simulink model "ModeleMachineInduction"  (R2022b)
settings: Solver=VariableStepAuto  StartTime=0.0  StopTime=10.0  MaxStep=10e-6  RelTol=1e-3
values from neighbouring files (symbols this model uses):
  fv = 0.08    [MotorDat_MSTPM1 (1).m]    (also in ParamMinduction0.m = 0.137399950871)
  h = 50e-6    (= 5e-05)    [MotorDat_MSTPM1 (1).m]    (also in ParamMinduction0.m; parametres.m = 1e-05)
  J = 0.004    [MotorDat_MSTPM1 (1).m]    (also in ParamMinduction0.m = 0.006; parametres.m = 0.000131)
  k_v = 0.8489    [ParamMinduction0.m]
  lcs_v = 62e-3    (= 0.062)    [ParamMinduction0.m]
  p = 4    [MotorDat_MSTPM1 (1).m]    (also in ParamMinduction0.m = 2)
  Rr_v = 1.8    [ParamMinduction0.m]
  Rs_v = 2.5    [ParamMinduction0.m]
  Tr_v = Lcr_v/Rr_v    (= 0.268333333333)    [ParamMinduction0.m]
  Vmax = 530    [MotorDat_MSTPM1 (1).m]    (also in ParamMinduction0.m = 650; parametres.m = 0.171666666667)
libraries: simulink x1, slpidlib x1
settings Model: Creator=dgrenier  LastModifiedBy=boris
settings DebuggingCC: UnconnectedInputMsg=warning  UnconnectedOutputMsg=warning  UnconnectedLineMsg=warning
settings ModelReferenceCC: EnableRefExpFcnMdlSchedulingChecks=on
settings RTWCC: DLArmComputeVersion=19.05

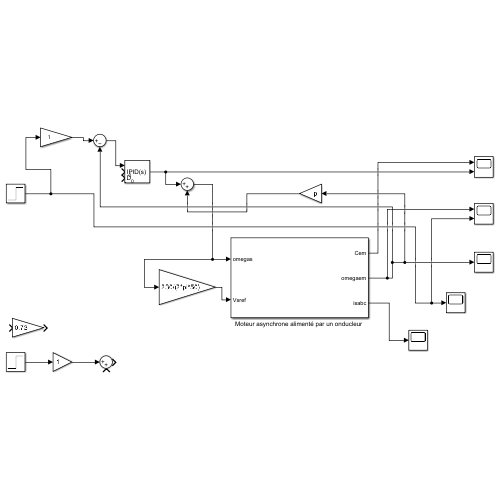
[thumbnail: Simulink's stored preview of the top-level diagram]
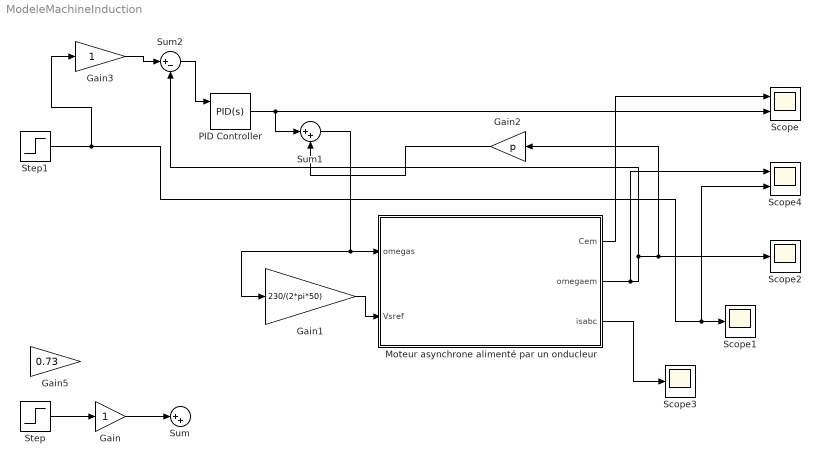
== system ModeleMachineInduction ==
  Gain : Gain
  Gain1 : Gain  Gain=230/(2*pi*50)
  Gain2 : Gain  Gain=p
  Gain3 : Gain
  Gain5 : Gain  Gain=0.73
  "Moteur asynchrone alimenté par un onducleur " : Subsystem
  PID Controller : slpidlib/PID Controller  Controller=PID  Form=Parallel  TimeDomain=Continuous-time  UseExternalTs=off  SampleTime=-1  IntegratorMethod=Forward Euler  FilterMethod=Forward Euler  ControllerParametersSource=internal  P=10  I=1  UseKiTs=off  D=0  N=100  UseFilter=on  TunerSelectOption=Transfer Function Based (PID Tuner App)  InitialConditionSource=external  InitialConditionForIntegrator=0  InitialConditionForFilter=0  DifferentiatorICPrevScaledInput=0  ExternalReset=none  TrackingMode=off  Kt=1  LimitOutput=off  SatLimitsSource=internal  UpperSaturationLimit=inf  LowerSaturationLimit=-inf  LinearizeAsGain=on  AntiWindupMode=none  Kb=1  LimitIntegrator=off  UpperIntegratorSaturationLimit=inf  LowerIntegratorSaturationLimit=-inf  POutMin=[]  POutMax=[]  IOutMin=[]  IOutMax=[]  DOutMin=[]  DOutMax=[]  NOutMin=[]  NOutMax=[]  SumOutMin=[]  SumOutMax=[]  SaturationOutMin=[]  SaturationOutMax=[]  PParamMin=[]  PParamMax=[]  IParamMin=[]  IParamMax=[]  DParamMin=[]  DParamMax=[]  NParamMin=[]  NParamMax=[]  KbParamMin=[]  KbParamMax=[]  KtParamMin=[]  KtParamMax=[]  KbOutMin=[]  KbOutMax=[]  KtOutMin=[]  KtOutMax=[]  IntegratorOutMin=[]  IntegratorOutMax=[]  FilterOutMin=[]  FilterOutMax=[]  SumI1OutMin=[]  SumI1OutMax=[]  SumI2OutMin=[]  SumI2OutMax=[]  SumI3OutMin=[]  SumI3OutMax=[]  SumI4OutMin=[]  SumI4OutMax=[]  SumDOutMin=[]  SumDOutMax=[]  DifferentiatorOutMin=[]  DifferentiatorOutMax=[]  FilterDiffOutCoefMin=[]  FilterDiffOutCoefMax=[]  ReciprocalOutMin=[]  ReciprocalOutMax=[]  SumDenOutMin=[]  SumDenOutMax=[]  SumNumOutMin=[]  SumNumOutMax=[]  DivideOutMin=[]  DivideOutMax=[]  UdiffTsProdOutMin=[]  UdiffTsProdOutMax=[]  NTsProdOutMin=[]  NTsProdOutMax=[]  UintegralTsProdOutMin=[]  UintegralTsProdOutMax=[]  UngainTsProdOutMin=[]  UngainTsProdOutMax=[]  ClampingZeroOutDataTypeStr=Inherit: Inherit via back propagation  ClampingZeroOutMin=[]  ClampingZeroOutMax=[]  FilterDenConstantOutDataTypeStr=Inherit: Inherit via back propagation  FilterDenConstantOutMin=[]  FilterDenConstantOutMax=[]  PCopyOutDataTypeStr=Inherit: Inherit via back propagation  PCopyOutMin=[]  PCopyOutMax=[]  NCopyOutDataTypeStr=Inherit: Inherit via back propagation  NCopyOutMin=[]  NCopyOutMax=[]  IntegratorContinuousStateAttributes=''  IntegratorStateMustResolveToSignalObject=off  IntegratorRTWStateStorageClass=Auto  FilterContinuousStateAttributes=''  FilterStateMustResolveToSignalObject=off  FilterRTWStateStorageClass=Auto  ParallelPVariant=InternalParameters  IdealPVariant=Disabled  IVariant=InternalParameters  DVariant=InternalParameters  IntegratorVariant=Continuous  SatVariant=Disabled  AWVariant=Passthrough  PCopyVariant=Disabled  TRVariant=Disabled  FdbkBlocksVariant=Forward  IdealPFdbkVariant=Disabled  SatFdbkVariant=Disabled  DerivativeFilterVariant=ContFilter  NVariant=InternalParameters  NCopyVariant=Disabled  FilterICVariant=ExternalICs  IntegratorICVariant=ExternalICs  ExternalResetVariant=Disabled  TRSumVariant=Passthrough  SumFdbkVariant=Disabled  SumVariant=Sum_PID  TsampFilterVariant=InternalTs  TsampNgainVariant=Passthrough  TsampIntegralVariant=Passthrough  ExternalSaturationOutDataTypeStr=Inherit: Same as second input
  Scope : Scope  NumInputPorts=2
  Scope1 : Scope
  Scope2 : Scope
  Scope3 : Scope
  Scope4 : Scope  NumInputPorts=2
  Step : Step  SampleTime=0
  Step1 : Step  After=10  SampleTime=1
  Sum : Sum  Inputs=|++
  Sum1 : Sum  Inputs=|++
  Sum2 : Sum  Inputs=|+-
  wires:
  Gain/1 -> Sum/1
  Step/1 -> Gain/1
  Sum1/1 -> Gain1/1, "Moteur asynchrone alimenté par un onducleur "/1(omegas)
  Gain2/1 -> Sum1/2
  "Moteur asynchrone alimenté par un onducleur "/2(omegaem) -> Scope4/1, Scope2/1, Gain2/1, Sum2/2
  "Moteur asynchrone alimenté par un onducleur "/3(isabc) -> Scope3/1
  Gain1/1 -> "Moteur asynchrone alimenté par un onducleur "/2(Vsref)
  Step1/1 -> Scope4/2, Scope1/1, Gain3/1
  Sum2/1 -> PID Controller/1
  Gain3/1 -> Sum2/1
  "Moteur asynchrone alimenté par un onducleur "/1(Cem) -> Scope/1
  PID Controller/1 -> Sum1/1, Scope/2

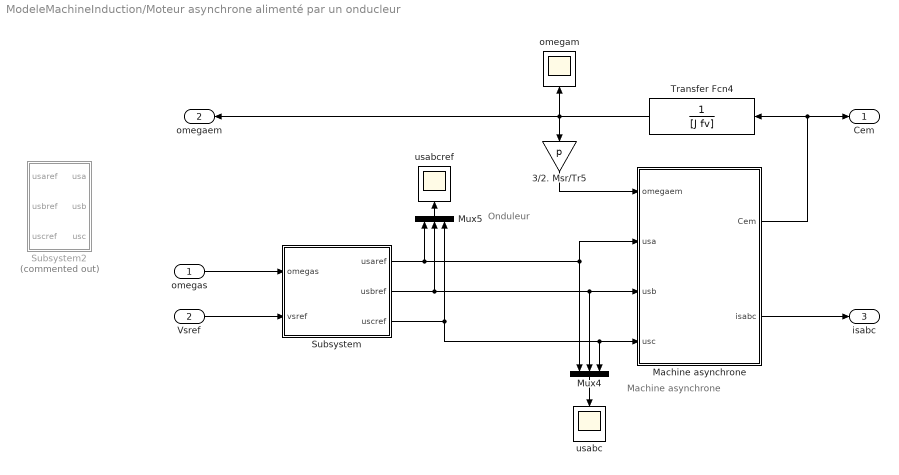
== system ModeleMachineInduction/Moteur asynchrone alimenté par un onducleur  ==
  note: Machine asynchrone
  note: Onduleur
  omegas : Inport
  Vsref : Inport  Port=2
  3/2. Msr/Tr5 : Gain  Gain=p
  Machine asynchrone : Subsystem
  Mux4 : Mux  Inputs=3
  Mux5 : Mux  Inputs=3
  Subsystem : Subsystem
  Subsystem2 : Subsystem  Commented=on
  Transfer Fcn4 : TransferFcn  Denominator=[J fv]
  "omegam " : Scope
  usabc : Scope
  usabcref : Scope
  Cem : Outport
  omegaem : Outport  Port=2
  isabc : Outport  Port=3
  wires:
  omegas/1 -> Subsystem/1(omegas)
  Vsref/1 -> Subsystem/2(vsref)
  Subsystem/3(uscref) -> Machine asynchrone/4(usc), Mux4/3, Mux5/3
  Subsystem/1(usaref) -> Machine asynchrone/2(usa), Mux4/1, Mux5/1
  Mux5/1 -> usabcref/1
  Subsystem/2(usbref) -> Machine asynchrone/3(usb), Mux4/2, Mux5/2
  Mux4/1 -> usabc/1
  Machine asynchrone/1(Cem) -> Cem/1, Transfer Fcn4/1
  Machine asynchrone/2(isabc) -> isabc/1
  3/2. Msr/Tr5/1 -> Machine asynchrone/1(omegaem)
  Transfer Fcn4/1 -> "omegam "/1, 3/2. Msr/Tr5/1, omegaem/1

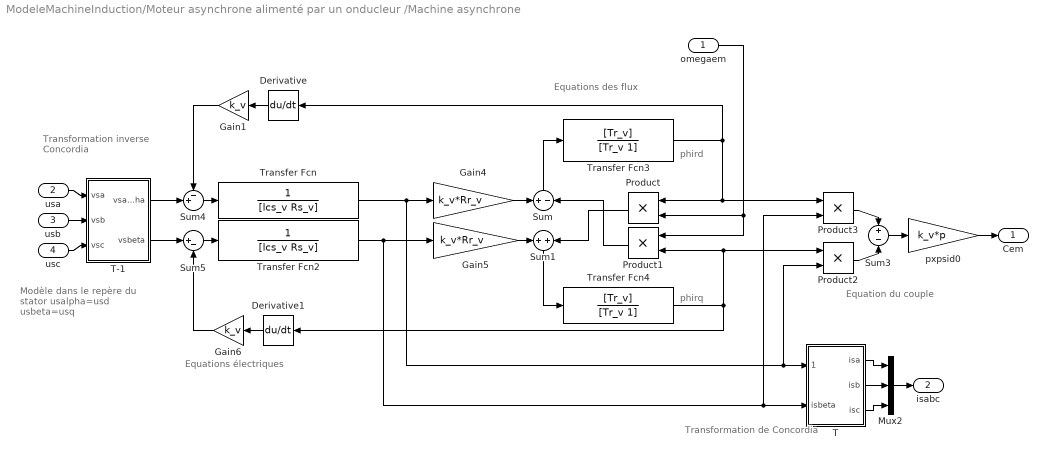
== system ModeleMachineInduction/Moteur asynchrone alimenté par un onducleur /Machine asynchrone ==
  note: Transformation
      | de Concordia
  note: Transformation
      | inverse Concordia
  note: Equation du couple
  note: Equations électriques
  note: Modèle dans le
      | repère du stator
      | usalpha=usd
      | usbeta=usq
  note: Equations des flux
  note: phird
  note: phirq
  omegaem : Inport
  usa : Inport  Port=2
  usb : Inport  Port=3
  usc : Inport  Port=4
  Derivative : Derivative
  Derivative1 : Derivative
  Gain1 : Gain  Gain=k_v
  Gain4 : Gain  Gain=k_v*Rr_v
  Gain5 : Gain  Gain=k_v*Rr_v
  Gain6 : Gain  Gain=k_v
  Mux2 : Mux  Inputs=3
  Product{,1..3} (4 alike) : Product  RndMeth=Zero
  Sum : Sum  Inputs=+|-
  Sum1 : Sum  Inputs=+|+
  Sum3 : Sum  Inputs=+|-
  Sum4 : Sum  Inputs=-+|
  Sum5 : Sum  Inputs=|+-
  T : Subsystem
  T-1 : Subsystem
  Transfer Fcn : TransferFcn  Denominator=[lcs_v Rs_v]
  Transfer Fcn2 : TransferFcn  Denominator=[lcs_v Rs_v]
  Transfer Fcn3 : TransferFcn  Numerator=[Tr_v]  Denominator=[Tr_v 1]
  Transfer Fcn4 : TransferFcn  Numerator=[Tr_v]  Denominator=[Tr_v 1]
  pxpsid0 : Gain  Gain=k_v*p
  Cem : Outport  VectorParamsAs1DForOutWhenUnconnected=off
  isabc : Outport  Port=2  VectorParamsAs1DForOutWhenUnconnected=off
  wires:
  Product2/1 -> Sum3/2
  Product3/1 -> Sum3/1
  Gain5/1 -> Sum1/1
  Gain4/1 -> Sum/1
  usc/1 -> T-1/3(vsc)
  usb/1 -> T-1/2(vsb)
  usa/1 -> T-1/1(vsa)
  Product1/1 -> Sum/2
  Product/1 -> Sum1/2
  T-1/2(vsbeta) -> Sum5/1
  T-1/1(vsalpha) -> Sum4/2
  Transfer Fcn/1 -> Gain4/1, Product2/2, T/1(isalpha)
  Transfer Fcn2/1 -> Gain5/1, Product3/2, T/2(isbeta)
  Sum/1 -> Transfer Fcn3/1
  Sum1/1 -> Transfer Fcn4/1
  Transfer Fcn3/1 -> Derivative/1, Product/1, Product3/1
  Transfer Fcn4/1 -> Product1/2, Product2/1, Derivative1/1
  omegaem/1 -> Product1/1, Product/2
  Gain6/1 -> Sum5/2
  Gain1/1 -> Sum4/1
  Sum3/1 -> pxpsid0/1
  pxpsid0/1 -> Cem/1
  Sum5/1 -> Transfer Fcn2/1
  Sum4/1 -> Transfer Fcn/1
  T/1(isa) -> Mux2/1
  T/2(isb) -> Mux2/2
  T/3(isc) -> Mux2/3
  Mux2/1 -> isabc/1
  Derivative/1 -> Gain1/1
  Derivative1/1 -> Gain6/1

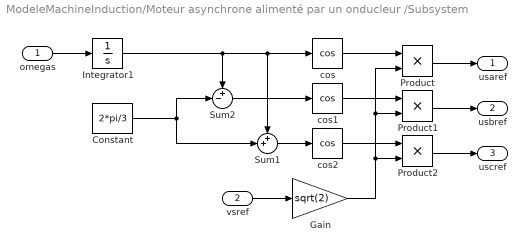
== system ModeleMachineInduction/Moteur asynchrone alimenté par un onducleur /Subsystem ==
  omegas : Inport
  vsref : Inport  Port=2
  Constant : Constant  Value=2*pi/3
  Gain : Gain  Gain=sqrt(2)
  Integrator1 : Integrator
  Product : Product  RndMeth=Zero
  Product1 : Product  RndMeth=Zero
  Product2 : Product  RndMeth=Zero
  Sum1 : Sum  Inputs=++|
  Sum2 : Sum  Inputs=+-|
  cos : Trigonometry  Operator=cos
  cos1 : Trigonometry  Operator=cos
  cos2 : Trigonometry  Operator=cos
  usaref : Outport
  usbref : Outport  Port=2
  uscref : Outport  Port=3
  wires:
  Product/1 -> usaref/1
  Product2/1 -> uscref/1
  Product1/1 -> usbref/1
  omegas/1 -> Integrator1/1
  cos/1 -> Product/1
  Integrator1/1 -> Sum1/1, cos/1, Sum2/1
  Constant/1 -> Sum1/2, Sum2/2
  Gain/1 -> Product/2, Product1/2, Product2/2
  vsref/1 -> Gain/1
  Sum2/1 -> cos1/1
  Sum1/1 -> cos2/1
  cos2/1 -> Product2/1
  cos1/1 -> Product1/1

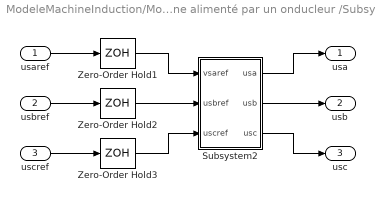
== system ModeleMachineInduction/Moteur asynchrone alimenté par un onducleur /Subsystem2 ==
  usaref : Inport
  usbref : Inport  Port=2
  uscref : Inport  Port=3
  Subsystem2 : Subsystem
  Zero-Order Hold1 : ZeroOrderHold  SampleTime=h
  Zero-Order Hold2 : ZeroOrderHold  SampleTime=h
  Zero-Order Hold3 : ZeroOrderHold  SampleTime=h
  usa : Outport  VectorParamsAs1DForOutWhenUnconnected=off
  usb : Outport  Port=2  VectorParamsAs1DForOutWhenUnconnected=off
  usc : Outport  Port=3  VectorParamsAs1DForOutWhenUnconnected=off
  wires:
  Zero-Order Hold1/1 -> Subsystem2/1(vsaref)
  Zero-Order Hold2/1 -> Subsystem2/2(usbref)
  Zero-Order Hold3/1 -> Subsystem2/3(uscref)
  uscref/1 -> Zero-Order Hold3/1
  usbref/1 -> Zero-Order Hold2/1
  usaref/1 -> Zero-Order Hold1/1
  Subsystem2/1(usa) -> usa/1
  Subsystem2/2(usb) -> usb/1
  Subsystem2/3(usc) -> usc/1

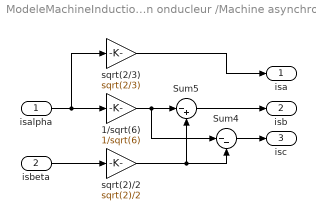
== system ModeleMachineInduction/Moteur asynchrone alimenté par un onducleur /Machine asynchrone/T ==
  isalpha : Inport
  isbeta : Inport  Port=2
  1/sqrt(6) : Gain  Gain=1/sqrt(6)
  Sum4 : Sum  Inputs=|--
  Sum5 : Sum  Inputs=|-+
  sqrt(2)/2 : Gain  Gain=sqrt(2)/2
  sqrt(2/3) : Gain  Gain=sqrt(2/3)
  isa : Outport  VectorParamsAs1DForOutWhenUnconnected=off
  isb : Outport  Port=2  VectorParamsAs1DForOutWhenUnconnected=off
  isc : Outport  Port=3  VectorParamsAs1DForOutWhenUnconnected=off
  wires:
  isbeta/1 -> sqrt(2)/2/1
  Sum4/1 -> isc/1
  Sum5/1 -> isb/1
  sqrt(2/3)/1 -> isa/1
  sqrt(2)/2/1 -> Sum4/2, Sum5/2
  1/sqrt(6)/1 -> Sum4/1, Sum5/1
  isalpha/1 -> 1/sqrt(6)/1, sqrt(2/3)/1

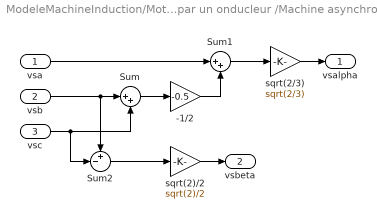
== system ModeleMachineInduction/Moteur asynchrone alimenté par un onducleur /Machine asynchrone/T-1 ==
  vsa : Inport
  vsb : Inport  Port=2
  vsc : Inport  Port=3
  -1/2 : Gain  Gain=-0.5
  Sum : Sum  Inputs=|++
  Sum1 : Sum  Inputs=|++
  Sum2 : Sum  Inputs=+-|
  sqrt(2)/2 : Gain  Gain=sqrt(2)/2
  sqrt(2/3) : Gain  Gain=sqrt(2/3)
  vsalpha : Outport  VectorParamsAs1DForOutWhenUnconnected=off
  vsbeta : Outport  Port=2  VectorParamsAs1DForOutWhenUnconnected=off
  wires:
  sqrt(2)/2/1 -> vsbeta/1
  sqrt(2/3)/1 -> vsalpha/1
  vsa/1 -> Sum1/1
  Sum2/1 -> sqrt(2)/2/1
  Sum1/1 -> sqrt(2/3)/1
  -1/2/1 -> Sum1/2
  Sum/1 -> -1/2/1
  vsc/1 -> Sum2/2, Sum/2
  vsb/1 -> Sum2/1, Sum/1

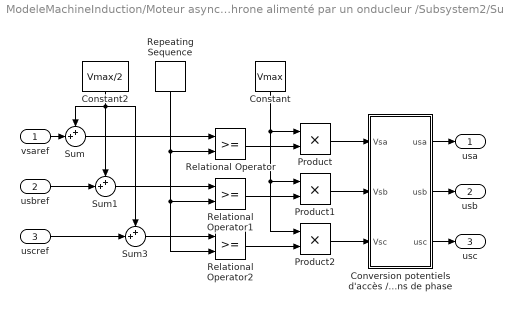
== system ModeleMachineInduction/Moteur asynchrone alimenté par un onducleur /Subsystem2/Subsystem2 ==
  vsaref : Inport
  usbref : Inport  Port=2
  uscref : Inport  Port=3
  Constant : Constant  Value=Vmax
  Constant2 : Constant  Value=Vmax/2
  Conversion potentiels d'accès / tensions de phase : Subsystem
  Product : Product  RndMeth=Zero
  Product1 : Product  RndMeth=Zero
  Product2 : Product  RndMeth=Zero
  Relational Operator : RelationalOperator  OutDataTypeStr=boolean  ZeroCross=off  InputSameDT=off
  Relational Operator1 : RelationalOperator  OutDataTypeStr=boolean  ZeroCross=off  InputSameDT=off
  Relational Operator2 : RelationalOperator  OutDataTypeStr=boolean  ZeroCross=off  InputSameDT=off
  Repeating Sequence : simulink/Sources/Repeating Sequence  rep_seq_t=[0 h/2 h]  rep_seq_y=[0 Vmax 0]
  Sum : Sum  Inputs=++|
  Sum1 : Sum  Inputs=++|
  Sum3 : Sum  Inputs=++|
  usa : Outport
  usb : Outport  Port=2
  usc : Outport  Port=3
  wires:
  Constant2/1 -> Sum3/1, Sum/1, Sum1/1
  Product2/1 -> Conversion potentiels d'accès / tensions de phase/3(Vsc)
  Product1/1 -> Conversion potentiels d'accès / tensions de phase/2(Vsb)
  Product/1 -> Conversion potentiels d'accès / tensions de phase/1(Vsa)
  Relational Operator2/1 -> Product2/2
  Sum3/1 -> Relational Operator2/1
  uscref/1 -> Sum3/2
  Sum1/1 -> Relational Operator1/1
  usbref/1 -> Sum1/2
  Sum/1 -> Relational Operator/1
  vsaref/1 -> Sum/2
  Relational Operator1/1 -> Product1/2
  Constant/1 -> Product2/1, Product1/1, Product/1
  Relational Operator/1 -> Product/2
  Repeating Sequence/1 -> Relational Operator2/2, Relational Operator1/2, Relational Operator/2
  Conversion potentiels d'accès / tensions de phase/3(usc) -> usc/1
  Conversion potentiels d'accès / tensions de phase/2(usb) -> usb/1
  Conversion potentiels d'accès / tensions de phase/1(usa) -> usa/1

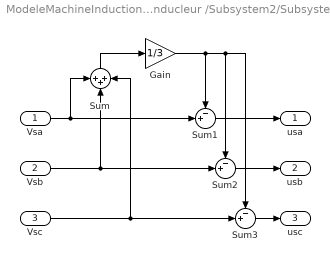
== system ModeleMachineInduction/Moteur asynchrone alimenté par un onducleur /Subsystem2/Subsystem2/Conversion potentiels d'accès // tensions de phase ==
  Vsa : Inport
  Vsb : Inport  Port=2
  Vsc : Inport  Port=3
  Gain : Gain  Gain=1/3
  Sum : Sum  Inputs=+++
  Sum1 : Sum  Inputs=-+|
  Sum2 : Sum  Inputs=-+|
  Sum3 : Sum  Inputs=-+|
  usa : Outport
  usb : Outport  Port=2
  usc : Outport  Port=3
  wires:
  Sum3/1 -> usc/1
  Sum2/1 -> usb/1
  Sum1/1 -> usa/1
  Gain/1 -> Sum3/1, Sum2/1, Sum1/1
  Sum/1 -> Gain/1
  Vsc/1 -> Sum/3, Sum3/2
  Vsb/1 -> Sum/2, Sum2/2
  Vsa/1 -> Sum/1, Sum1/2
